simulink model "Mesh_4Node_1BaseStation_System"  (R2024b)
settings: Solver=FixedStepAuto  StartTime=0.0  StopTime=210  FixedStep=1  RelTol=1e-3
settings Model: Creator=ARYA MGC  LastModifiedBy=ARYA MGC

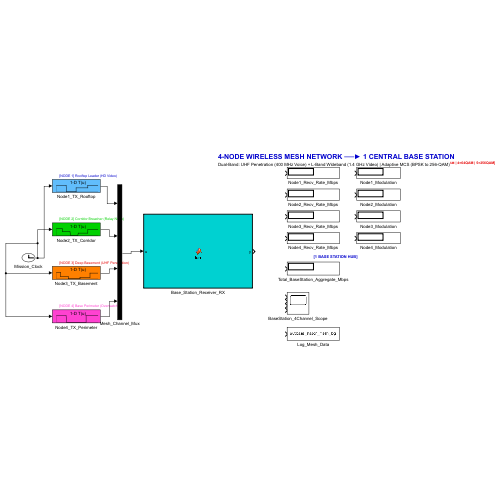
[thumbnail: Simulink's stored preview of the top-level diagram]
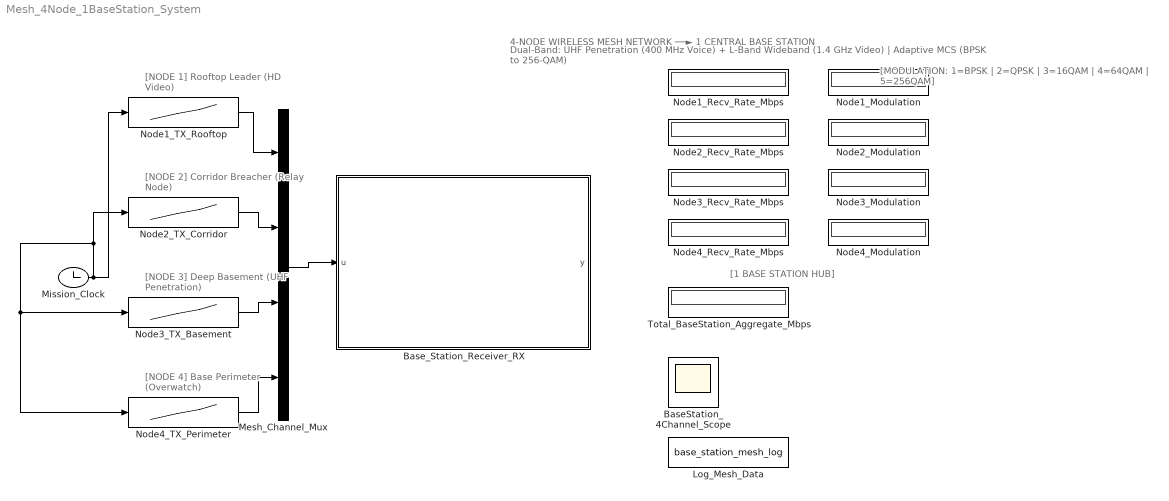
== system Mesh_4Node_1BaseStation_System ==
  note: 4-NODE WIRELESS MESH NETWORK ──► 1 CENTRAL BASE STATION
  note: Dual-Band: UHF Penetration (400 MHz Voice) + L-Band Wideband (1.4 GHz Video) | Adaptive MCS (BPSK to 256-QAM)
  note: [NODE 1] Rooftop Leader (HD Video)
  note: [NODE 2] Corridor Breacher (Relay Node)
  note: [NODE 3] Deep Basement (UHF Penetration)
  note: [NODE 4] Base Perimeter (Overwatch)
  note: [1 BASE STATION HUB]
  note: [MODULATION: 1=BPSK | 2=QPSK | 3=16QAM | 4=64QAM | 5=256QAM]
  BaseStation_4Channel_Scope : Scope  NumInputPorts=4
  Base_Station_Receiver_RX : MATLAB Function  TreatAsAtomicUnit=on
  Log_Mesh_Data : ToWorkspace  VariableName=base_station_mesh_log  SampleTime=-1
  Mesh_Channel_Mux : Mux
  Mission_Clock : Clock
  Node1_Modulation : Display
  Node1_Recv_Rate_Mbps : Display
  Node1_TX_Rooftop : Lookup_n-D  NumberOfTableDimensions=1  BreakpointsForDimension1=[0 50 51 100 101 160 161 210]  Table=[30 30 18 18 25 25 30 30]  InternalRulePriority=Speed  RndMeth=Simplest
  Node2_Modulation : Display
  Node2_Recv_Rate_Mbps : Display
  Node2_TX_Corridor : Lookup_n-D  NumberOfTableDimensions=1  BreakpointsForDimension1=[0 30 31 70 71 110 111 160 161 210]  Table=[22 22 15 15 8 8 12 12 20 20]  InternalRulePriority=Speed  RndMeth=Simplest
  Node3_Modulation : Display
  Node3_Recv_Rate_Mbps : Display
  Node3_TX_Basement : Lookup_n-D  NumberOfTableDimensions=1  BreakpointsForDimension1=[0 20 21 60 61 120 121 170 171 210]  Table=[20 20 10 10 5 5 8 8 18 18]  InternalRulePriority=Speed  RndMeth=Simplest
  Node4_Modulation : Display
  Node4_Recv_Rate_Mbps : Display
  Node4_TX_Perimeter : Lookup_n-D  NumberOfTableDimensions=1  BreakpointsForDimension1=[0 50 51 150 151 210]  Table=[25 25 20 20 25 25]  InternalRulePriority=Speed  RndMeth=Simplest
  Total_BaseStation_Aggregate_Mbps : Display
  wires:
  Mission_Clock/1 -> Node4_TX_Perimeter/1, Node3_TX_Basement/1, Node2_TX_Corridor/1, Node1_TX_Rooftop/1
  Node1_TX_Rooftop/1 -> Mesh_Channel_Mux/1
  Node2_TX_Corridor/1 -> Mesh_Channel_Mux/2
  Node3_TX_Basement/1 -> Mesh_Channel_Mux/3
  Node4_TX_Perimeter/1 -> Mesh_Channel_Mux/4
  Mesh_Channel_Mux/1 -> Base_Station_Receiver_RX/1(u)

== matlab function Mesh_4Node_1BaseStation_System/Base_Station_Receiver_RX ==
  data: u input; y output
function y = fcn(u)

y = u;
